simulink model "openloopresponce"  (R2020b)
settings: Solver=VariableStepAuto  StartTime=0.0  StopTime=10  RelTol=1e-3
settings Model: Creator=Altay  LastModifiedBy=Altay

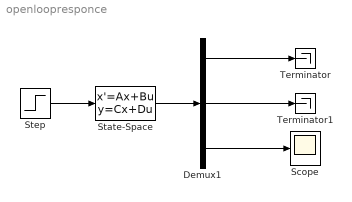
== system openloopresponce ==
  Demux1 : Demux  Outputs=3
  "Scope " : Scope
  "State-Space " : StateSpace  A=[-0.313 56.7 0; -0.0139 -0.426 0; 0 56.7 0]  B=[0.232; 0.0203; 0]  C=eye(3)  D=[0; 0; 0]  InitialCondition=0  ContinuousStateAttributes={'Hamle_acisi','Pitch_orani','Pitch_acisi'}
  "Step " : Step  Time=0  After=0.2  SampleTime=0
  "Terminator " : Terminator
  "Terminator1 " : Terminator
  wires:
  Demux1/1 -> "Terminator "/1
  Demux1/2 -> "Terminator1 "/1
  "State-Space "/1 -> Demux1/1
  "Step "/1 -> "State-Space "/1
  Demux1/3 -> "Scope "/1
